simulink model "week_1_springmass_systemmodel_classdemo"  (R2020b)
settings: Solver=VariableStepAuto  StartTime=0.0  StopTime=Sim_Time  RelTol=1e-3
undefined symbols (not defined in the file): b, k, m
settings Model: Creator=anime  LastModifiedBy=anime

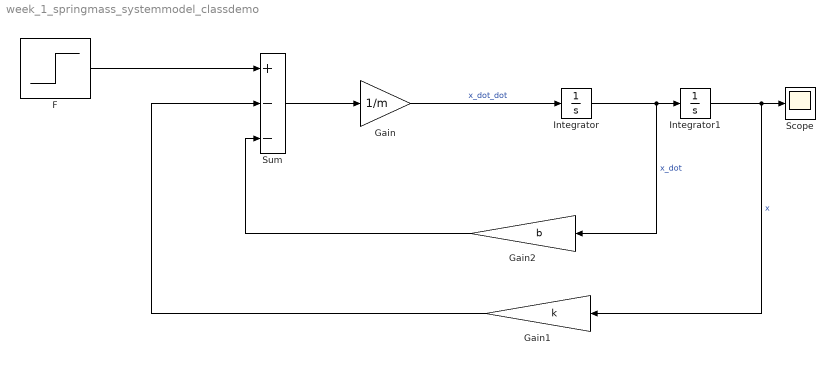
== system week_1_springmass_systemmodel_classdemo ==
  F : Step  After=2  SampleTime=0
  Gain : Gain  Gain=1/m
  Gain1 : Gain  Gain=k
  Gain2 : Gain  Gain=b
  Integrator : Integrator
  Integrator1 : Integrator
  Scope : Scope
  Sum : Sum  Inputs=+--
  wires:
  F/1 -> Sum/1
  Sum/1 -> Gain/1
  Gain/1 -> Integrator/1  "x_dot_dot"
  Integrator/1 -> Gain2/1, Integrator1/1  "x_dot"
  Integrator1/1 -> Gain1/1, Scope/1  "x"
  Gain1/1 -> Sum/2
  Gain2/1 -> Sum/3
